simulink model "kinematik_model"  (Simulink 8.4)
settings: Solver=ode45  StartTime=0.0  StopTime=10.0  RelTol=1e-3
libraries: simulink x1
settings Model: Creator=user  LastModifiedBy=DELL
settings DataIOCC: SignalLoggingSaveFormat=Dataset
settings OptimizationCC: ExpressionDepthLimit=128
settings DebuggingCC: FcnCallInpInsideContextMsg=EnableAllAsError
settings GRTTargetCC: CombineOutputUpdateFcns=on  GRTInterface=off

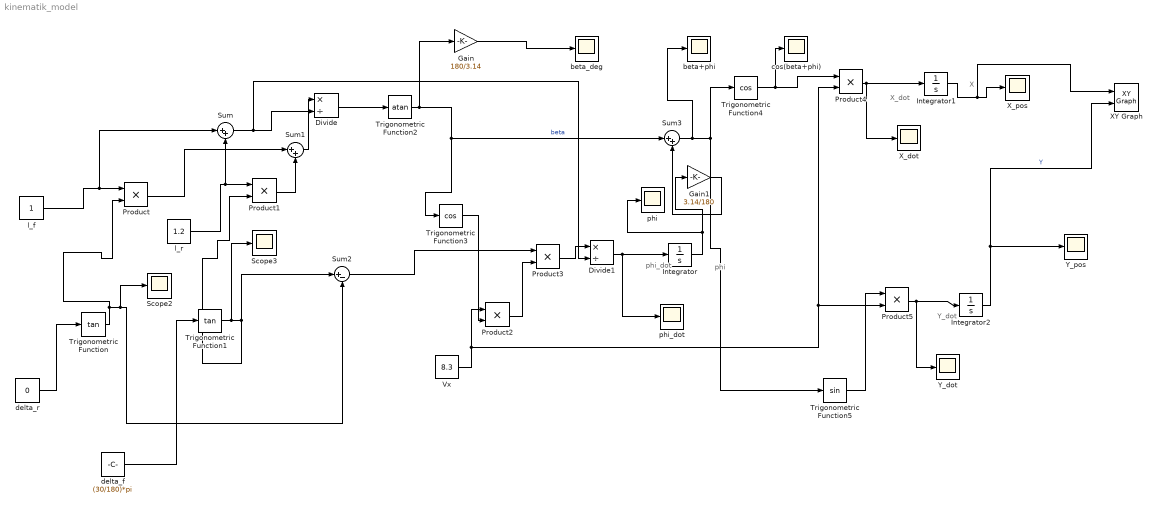
== system kinematik_model ==
  note: X
  note: Y_dot
  note: X_dot
  note: phi
  note: phi_dot
  Divide : Product  Inputs=*/
  Divide1 : Product  Inputs=*/
  Gain : Gain  Gain=180/3.14
  Gain1 : Gain  Gain=3.14/180
  Integrator : Integrator
  Integrator1 : Integrator
  Integrator2 : Integrator
  Product{,1..5} (6 alike) : Product
  Scope2 : Scope
      settings: SaveName=ScopeData2
  Scope3 : Scope
      settings: SaveName=ScopeData3
  Sum : Sum  Inputs=|++
  Sum1 : Sum  Inputs=|++
  Sum2 : Sum  Inputs=|+-
  Sum3 : Sum  Inputs=|++
  Trigonometric Function : Trigonometry  Operator=tan
  Trigonometric Function1 : Trigonometry  Operator=tan
  Trigonometric Function2 : Trigonometry  Operator=atan
  Trigonometric Function3 : Trigonometry  Operator=cos
  Trigonometric Function4 : Trigonometry  Operator=cos
  Trigonometric Function5 : Trigonometry
  Vx : Constant  Value=8.3
  XY Graph : simulink/Sinks/XY Graph  xmin=0  xmax=1000  ymin=0  ymax=1000  st=-1
  X_dot : Scope
      settings: SaveName=ScopeData4
  X_pos : Scope
  Y_dot : Scope
      settings: SaveName=ScopeData5
  Y_pos : Scope
  beta+phi : Scope
      settings: SaveName=ScopeData10
  beta_deg : Scope
      settings: SaveName=ScopeData6
  cos(beta+phi) : Scope
      settings: SaveName=ScopeData9
  delta_f : Constant  Value=(30/180)*pi
  delta_r : Constant  Value=0
  l_f : Constant
  l_r : Constant  Value=1.2
  phi : Scope
      settings: SaveName=ScopeData8
  phi_dot : Scope
      settings: SaveName=ScopeData7
  wires:
  delta_f/1 -> Trigonometric Function1/1
  delta_r/1 -> Trigonometric Function/1
  Trigonometric Function/1 -> Scope2/1, Sum2/2, Product/2
  Trigonometric Function1/1 -> Scope3/1, Product1/2, Sum2/1
  l_f/1 -> Sum/1, Product/1
  l_r/1 -> Sum/2, Product1/1
  Product/1 -> Sum1/1
  Product1/1 -> Sum1/2
  Sum1/1 -> Divide/1
  Sum/1 -> Divide1/2, Divide/2
  Divide/1 -> Trigonometric Function2/1
  Trigonometric Function2/1 -> Gain/1, Sum3/1, Trigonometric Function3/1  "beta"
  Sum2/1 -> Product3/1
  Vx/1 -> Product4/2, Product5/2, Product2/1
  Trigonometric Function3/1 -> Product2/2
  Product2/1 -> Product3/2
  Product3/1 -> Divide1/1
  Divide1/1 -> phi_dot/1, Integrator/1
  Integrator/1 -> Gain1/1, phi/1
  Sum3/1 -> beta+phi/1, Trigonometric Function4/1, Trigonometric Function5/1
  Trigonometric Function4/1 -> cos(beta+phi)/1, Product4/1
  Product4/1 -> X_dot/1, Integrator1/1
  Trigonometric Function5/1 -> Product5/1
  Product5/1 -> Y_dot/1, Integrator2/1
  Integrator1/1 -> XY Graph/1, X_pos/1
  Integrator2/1 -> XY Graph/2, Y_pos/1  "Y"
  Gain/1 -> beta_deg/1
  Gain1/1 -> Sum3/2
